simulink model "v2021_10_27_modello_calcolo_trim_1"  (R2020b)
settings: Solver=ode4  StartTime=0.0  StopTime=10  FixedStep=0.01  RelTol=1e-3
values from neighbouring files (symbols this model uses):
  alphavec_rad = [-0.10471975512 -0.0872664625997 -0.0698131700798 -0.0523598775598 -0.0349065850399 -0.0174532925199 0 0.0174532925199 0.0349065850399 0.0523598775598 0.0698131700798 0.0872664625997 ... (13 elements, 1x13)]    [datiAerodinamiciAENEA.mat]    (also in v2021_10_27_calcoloAerodinamica.m = deg2rad(alphavec))
  b = 2.62    [datiAerodinamiciAENEA.mat]    (also in derivateROSKAM_new.m; v2021_10_27_calcoloAerodinamica.m)
  betavec_rad = [-0.209439510239 -0.13962634016 -0.0698131700798 0 0.0698131700798 0.13962634016 0.209439510239]    [datiAerodinamiciAENEA.mat]    (also in v2021_10_27_calcoloAerodinamica.m = deg2rad(betavec))
  c = 0.32    [datiAerodinamiciAENEA.mat]    (also in derivateROSKAM_new.m; v2021_10_27_calcoloAerodinamica.m)
  cbar = 0.32    [datiAerodinamiciAENEA.mat]    (also in v2021_10_27_calcoloAerodinamica.m)
  CD0 = 0.2    [datiAerodinamiciAENEA.mat]    (also in v2021_10_27_calcoloAerodinamica.m = 0.024)
  CldA = KCldA(1)*180/pi    [Alettoni.m]    (also in datiAerodinamiciAENEA.mat = 0.490103315517)
  CLdE = KCLdE(1)*180/pi    [Equilibratore.m]    (also in datiAerodinamiciAENEA.mat = 0.809101149087)
  CldR = 0.0568697125654    [datiAerodinamiciAENEA.mat]
  Clp = -0.4318    [datiAerodinamiciAENEA.mat]    (also in derivateROSKAM_new.m = clp_w+2*(Zv/b)^2*cy_betav+Clp_tail; v2021_10_27_calcoloAerodinamica.m)
  CLq = 8.13    [datiAerodinamiciAENEA.mat]    (also in v2021_10_27_calcoloAerodinamica.m)
  Clr = 0.1459    [datiAerodinamiciAENEA.mat]    (also in derivateROSKAM_new.m = cl*clr_cl-(2/b^2)*(lv*cos(alpha)+Zv*sin(alpha))*(Zv*cos(alph; v2021_10_27_calcoloAerodinamica.m)
  CmdE = KCmdE(1)*180/pi    [Equilibratore.m]    (also in datiAerodinamiciAENEA.mat = -3.59730623976)
  Cmq = -23.24    [datiAerodinamiciAENEA.mat]    (also in derivateROSKAM_new.m = -K*cL_alphaw*((AR*(2*(Xw/c)^2+0.5*(Xw/c))/(AR+2))+1/8)-2*cL_; v2021_10_27_calcoloAerodinamica.m)
  CndA = KCndA(1)*180/pi    [Alettoni.m]    (also in datiAerodinamiciAENEA.mat = -0.0456969018066)
  CndR = -0.162544523826    [datiAerodinamiciAENEA.mat]
  Cnp = 0.000294    [datiAerodinamiciAENEA.mat]    (also in derivateROSKAM_new.m = -clp_w*tan(alpha)+Clp*tan(alpha)-(2/b)*(lv*cos(alpha)+Zv*sin; v2021_10_27_calcoloAerodinamica.m = 0.007507)
  Cnr = -0.4872    [datiAerodinamiciAENEA.mat]    (also in derivateROSKAM_new.m = (Cnr_Clquadro)*cl^2+(cnr_cd0)*cd0+(2/b^2)*(lv*cos(alpha)+Zv*; v2021_10_27_calcoloAerodinamica.m)
  CYdA = KCYdA(1)*180/pi    [Alettoni.m]    (also in datiAerodinamiciAENEA.mat = -0.0146577407549)
  CYdR = -0.298131751664    [datiAerodinamiciAENEA.mat]
  CYp = 0.050728    [datiAerodinamiciAENEA.mat]    (also in v2021_10_27_calcoloAerodinamica.m)
  CYr = 0.358925    [datiAerodinamiciAENEA.mat]    (also in v2021_10_27_calcoloAerodinamica.m)
  deltaAtrim = 0    [v2021_10_27_avvioSITL.m]
  deltaEtrim = (Cm0*CL_alpharad+Cm_alpharad*CLtrim)/(CL_alpharad*CmdE)    [calcoloDatiIniziali.m]    (also in v2021_10_27_avvioSITL.m = 0)
  deltaRtrim = 0    [v2021_10_27_avvioSITL.m]
  deltaTtrim = 0.1    [v2021_10_27_avvioSITL.m]
  Dprop = 0.5334    [datiAerodinamiciAENEA.mat]    (also in v2021_10_27_calcoloAerodinamica.m)
  J_vec = [0 0.03 0.06 0.09 0.11 0.14 0.17 0.2 0.23 0.26 0.28 0.31 ... (30 elements, 30x1)]    [datiAerodinamiciAENEA.mat]
  Jeng = 0    [datiAerodinamiciAENEA.mat]    (also in v2021_10_27_calcoloAerodinamica.m)
  Jprop = 0.00422031414    [datiAerodinamiciAENEA.mat]    (also in v2021_10_27_calcoloAerodinamica.m)
  q = prediction(11)    [f_pred_F1B.m]
  r = prediction(12)    [f_pred_F1B.m]
  rACtG = [-1.334 0 -0.2103]    [datiAerodinamiciAENEA.mat]    (also in v2021_10_27_calcoloAerodinamica.m = rACtP-rGP)
  rACwG = [-0.0589 0 -0.1645]    [datiAerodinamiciAENEA.mat]    (also in v2021_10_27_calcoloAerodinamica.m = rACwP-rGP)
  rAHRSG = [0 0 0.1075]    [datiAerodinamiciAENEA.mat]    (also in v2021_10_27_calcoloAerodinamica.m = rAHRSP-rGP)
  rho = 1.2133    [datiAerodinamiciAENEA.mat]    (also in derivateROSKAM_new.m = 1.16123787958; v2021_10_27_calcoloAerodinamica.m)
  rLEG = [0.0211 0 -0.1645]    [datiAerodinamiciAENEA.mat]    (also in v2021_10_27_calcoloAerodinamica.m = rLEP-rGP)
  rmglG = [-0.2319 -0.2 0.3925]    [datiAerodinamiciAENEA.mat]    (also in v2021_10_27_calcoloAerodinamica.m = rmglP-rGP)
  rmgrG = [-0.2319 0.2 0.3925]    [datiAerodinamiciAENEA.mat]    (also in v2021_10_27_calcoloAerodinamica.m = rmgrP-rGP)
  rngG = [0.2969 0 0.3925]    [datiAerodinamiciAENEA.mat]    (also in v2021_10_27_calcoloAerodinamica.m = rngP-rGP)
  rNPG = [-0.2442 0 -0.1645]    [datiAerodinamiciAENEA.mat]    (also in v2021_10_27_calcoloAerodinamica.m = rNPP-rGP)
  rPG = [0.5 0 -0.1075]    [datiAerodinamiciAENEA.mat]    (also in v2021_10_27_calcoloAerodinamica.m = -rGP)
  Rprop = 0.2667    [datiAerodinamiciAENEA.mat]    (also in v2021_10_27_calcoloAerodinamica.m)
  S = 0.8384    [datiAerodinamiciAENEA.mat]    (also in derivateROSKAM_new.m; v2021_10_27_calcoloAerodinamica.m)
  W = [0 0 92.214]    [datiAerodinamiciAENEA.mat]    (also in derivateROSKAM_new.m = 112.815; v2021_10_27_calcoloAerodinamica.m = m*g)
  Zeng = -0.1075    [datiAerodinamiciAENEA.mat]    (also in v2021_10_27_calcoloAerodinamica.m = rPG(3))
undefined symbols (not defined in the file or in its folder): F, matricepolinomi, MIL
libraries: aerolibwind2 x3, simulink x2, shared6dof x1, aerolibasang x1, pid_lib x1
(part 2 of 2)

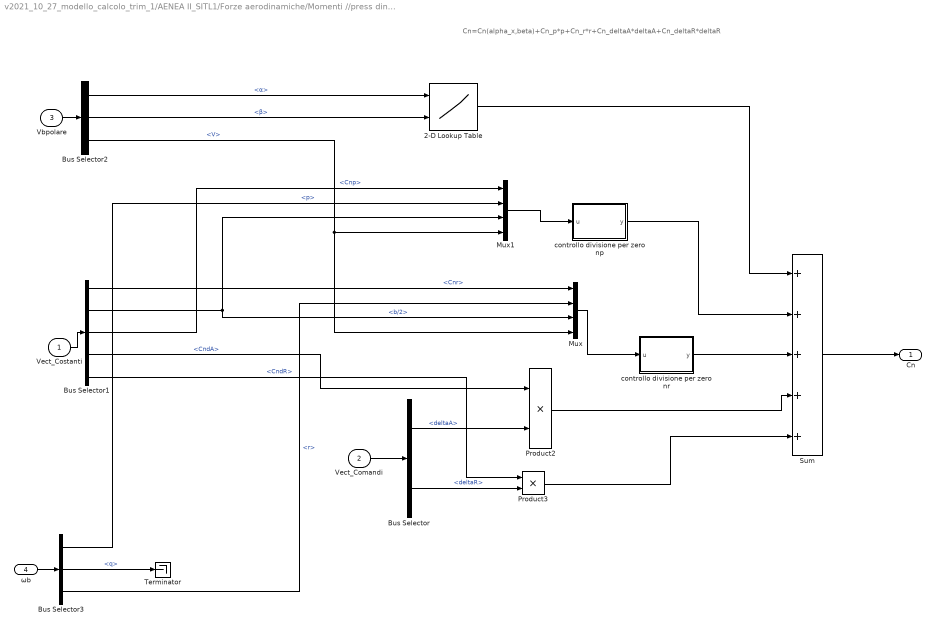
== system v2021_10_27_modello_calcolo_trim_1/AENEA II_SITL1/Forze aerodinamiche/Momenti //press din/Subsystem5 ==
  note: Cn=Cn(alpha_x,beta)+Cn_p*p+Cn_r*r+Cn_deltaA*deltaA+Cn_deltaR*deltaR
  Vect_Costanti : Inport
  Vect_Comandi : Inport  Port=2
  "Vbpolare " : Inport  Port=3
  ωb : Inport  Port=4
  2-D Lookup Table : Lookup_n-D  BreakpointsForDimension1=alphavec_rad  BreakpointsForDimension2=betavec_rad  Table=Cn(2:end,2:end)  InternalRulePriority=Speed  RndMeth=Simplest  InputSameDT=on
      settings: InputPortMap=u0,u1
  Bus Selector : BusSelector  OutputSignals=deltaA,deltaR
  Bus Selector1 : BusSelector  OutputSignals=Coef_Aerodinamici.Coef_Momenti.Cnr,Coef_Geometrici.b/2,Coef_Aerodinamici.Coef_Momenti.Cnp,Coef_Aerodinamici.Coef_Momenti.CndA,Coef_Aerodinamici.Coef_Momenti.CndR
  Bus Selector2 : BusSelector  OutputSignals=α,β,V
  Bus Selector3 : BusSelector  OutputSignals=p,q,r
  Mux : Mux
  Mux1 : Mux
  Product2 : Product
  Product3 : Product
  Sum : Sum  Inputs=5
  Terminator : Terminator
  "controllo divisione per zero np " : MATLAB Function  TreatAsAtomicUnit=on
  "controllo divisione per zero nr " : MATLAB Function  TreatAsAtomicUnit=on
  Cn : Outport  VectorParamsAs1DForOutWhenUnconnected=off
  wires:
  Bus Selector1/3 -> Mux1/1  "<Cnp>"
  Product2/1 -> Sum/4
  Product3/1 -> Sum/5
  Sum/1 -> Cn/1
  Bus Selector1/1 -> Mux/1  "<Cnr>"
  Bus Selector1/5 -> Product3/1  "<CndR>"
  Bus Selector/2 -> Product3/2  "<deltaR>"
  Bus Selector/1 -> Product2/2  "<deltaA>"
  2-D Lookup Table/1 -> Sum/1
  Vect_Comandi/1 -> Bus Selector/1
  Vect_Costanti/1 -> Bus Selector1/1
  Bus Selector1/4 -> Product2/1  "<CndA>"
  Bus Selector1/2 -> Mux1/3, Mux/3  "<b/2>"
  Bus Selector2/3 -> Mux1/4, Mux/4  "<V>"
  "Vbpolare "/1 -> Bus Selector2/1
  Bus Selector2/1 -> 2-D Lookup Table/1  "<α>"
  Bus Selector2/2 -> 2-D Lookup Table/2  "<β>"
  ωb/1 -> Bus Selector3/1
  Bus Selector3/3 -> Mux/2  "<r>"
  Bus Selector3/1 -> Mux1/2  "<p>"
  Bus Selector3/2 -> Terminator/1  "<q>"
  Mux/1 -> "controllo divisione per zero nr "/1(u)
  "controllo divisione per zero nr "/1(y) -> Sum/3
  Mux1/1 -> "controllo divisione per zero np "/1(u)
  "controllo divisione per zero np "/1(y) -> Sum/2

== matlab function v2021_10_27_modello_calcolo_trim_1/AENEA II_SITL1/Velocità1/MATLAB Function ==
  data: V input; module output
function module = absolute(V)

module=sqrt((V(1)^2)+(V(2)^2)+(V(3)^2));

end

== matlab function v2021_10_27_modello_calcolo_trim_1/AENEA II_SITL1/Velocità1/controllo divisione per 0 su alpha ==
  data: u input; y output
function y = tgalpha(u)

if length(u)~=2
    error('vettore ingresso errato')
else
    if u(2)==0
        y=0;
    else 
        y=u(1)/u(2);
    end
end

== matlab function v2021_10_27_modello_calcolo_trim_1/AENEA II_SITL1/Velocità1/controllo divisione per 0 su beta ==
  data: u input; y output
function y = sinbeta(u)

if length(u)~=2
    error('vettore ingresso errato')
else
    if u(2)==0
        y=0;
    else 
        y=u(1)/u(2);
    end
end

== matlab function v2021_10_27_modello_calcolo_trim_1/AENEA II_SITL1/Velocità1/MATLAB Function1 ==
  data: V input; module output
function module = absolute(V)

module=sqrt((V(1)^2)+(V(2)^2)+(V(3)^2));

end

== matlab function v2021_10_27_modello_calcolo_trim_1/AENEA II_SITL1/Forze aerodinamiche/Forze assi vento//q/Subsystem1/controllo divisione per zero Yp  ==
  data: u input; y output
function y = Yp(u)

if length(u)~=4
    error('vettore ingresso dimensione errata')
else
    if u(4)==0
        y=0;
    else
        y=u(1)*u(2)*u(3)/u(4);
    end
end

== matlab function v2021_10_27_modello_calcolo_trim_1/AENEA II_SITL1/Forze aerodinamiche/Forze assi vento//q/Subsystem1/controllo divisione per zero Yr ==
  data: u input; y output
function y = Yr(u)

if length(u)~=4
    error('vettore ingresso dimensione errata')
else
    if u(4)==0
        y=0;
    else
        y=u(1)*u(2)*u(3)/u(4);
    end
end

== matlab function v2021_10_27_modello_calcolo_trim_1/AENEA II_SITL1/Forze aerodinamiche/Forze assi vento//q/Subsystem2/controllo divisione per zero Lq  ==
  data: u input; y output
function y = Lq(u)

if length(u)~=4
    error('vettore ingresso dimensione errata')
else
    if u(4)==0
        y=0;
    else
        y=u(1)*u(2)*u(3)/u(4);
    end
end

== matlab function v2021_10_27_modello_calcolo_trim_1/AENEA II_SITL1/Forze aerodinamiche/MATLAB Function ==
  data: alpha input; Lbw output; beta input
function Lbw = DCMbw(alpha,beta)


Lbw=[cos(alpha)*cos(beta), -cos(alpha)*sin(beta), -sin(alpha); sin(beta), cos(beta), 0; sin(alpha)*cos(beta), -sin(alpha)*sin(beta), cos(alpha)];

== matlab function v2021_10_27_modello_calcolo_trim_1/AENEA II_SITL1/Forze aerodinamiche/Momenti //press din/Subsystem3/controllo divisione per zero lp  ==
  data: u input; y output
function y = lp(u)

if length(u)~=4
    error('vettore ingresso dimensione errata')
else
    if u(4)==0
        y=0;
    else
        y=u(1)*u(2)*u(3)/u(4);
    end
end

== matlab function v2021_10_27_modello_calcolo_trim_1/AENEA II_SITL1/Forze aerodinamiche/Momenti //press din/Subsystem3/controllo divisione per zero lr  ==
  data: u input; y output
function y = lr(u)

if length(u)~=4
    error('vettore ingresso dimensione errata')
else
    if u(4)==0
        y=0;
    else
        y=u(1)*u(2)*u(3)/u(4);
    end
end

== matlab function v2021_10_27_modello_calcolo_trim_1/AENEA II_SITL1/Forze aerodinamiche/Momenti //press din/Subsystem4/controllo divisione per zero mq  ==
  data: u input; y output
function y = mq(u)

if length(u)~=4
    error('vettore ingresso dimensione errata')
else
    if u(4)==0
        y=0;
    else
        y=u(1)*u(2)*u(3)/u(4);
    end
end

== matlab function v2021_10_27_modello_calcolo_trim_1/AENEA II_SITL1/Forze aerodinamiche/Momenti //press din/Subsystem5/controllo divisione per zero np  ==
  data: u input; y output
function y = np(u)

if length(u)~=4
    error('vettore ingresso dimensione errata')
else
    if u(4)==0
        y=0;
    else
        y=u(1)*u(2)*u(3)/u(4);
    end
end

== matlab function v2021_10_27_modello_calcolo_trim_1/AENEA II_SITL1/Forze aerodinamiche/Momenti //press din/Subsystem5/controllo divisione per zero nr  ==
  data: u input; y output
function y = nr(u)

if length(u)~=4
    error('vettore ingresso dimensione errata')
else
    if u(4)==0
        y=0;
    else
        y=u(1)*u(2)*u(3)/u(4);
    end
end

== matlab function v2021_10_27_modello_calcolo_trim_1/AENEA II_SITL1/MATLAB Function ==
  data: PHI input; invR output
function invR = omega2PHIdot(PHI)

if length(PHI)==3
    Phi=PHI(1);
    Theta=PHI(2);
    
    invR=[1, sin(Phi)*tan(Theta), cos(Phi)*tan(Theta); 0, cos(Phi), -sin(Phi); 0, sin(Phi)*sec(Theta), cos(Phi)*sec(Theta)];
else 
    error('il vettore PHI non va bene')
end

== matlab function v2021_10_27_modello_calcolo_trim_1/AENEA II_SITL1/Propulsione1/LUT ELICA /MATLAB Function ==
  data: J input; Ct output; RPM input; Cp output; matricepolinomi input
function [Ct,Cp] = calcolo_Ct_Cp(J,RPM,matricepolinomi)

lct00 = matricepolinomi(1,1);
lct10 = matricepolinomi(1,2);
lct01 = matricepolinomi(1,3);
lct20 = matricepolinomi(1,4);
lct11 = matricepolinomi(1,5);
lct02 = matricepolinomi(1,6);
lct30 = matricepolinomi(1,7);
lct21 = matricepolinomi(1,8);
lct12 = matricepolinomi(1,9);
lct40 = matricepolinomi(1,10);
lct31 = matricepolinomi(1,11);
lct22 = matricepolinomi(1,12);

qct00 = matricepolinomi(2,1);
qct10 = matricepolinomi(2,2);
qct01 = matricepolinomi(2,3);
qct20 = matricepolinomi(2,4);
qct11 = matricepolinomi(2,5);
qct02 = matricepolinomi(2,6);
qct30 = matricepolinomi(2,7);
qct21 = matricepolinomi(2,8);
qct12 = matricepolinomi(2,9);
qct03 = matricepolinomi(2,10);
qct40 = matricepolinomi(2,11);
qct31 = matricepolinomi(2,12);
qct22 = matricepolinomi(2,13);
qct13 = matricepolinomi(2,14);
qct04 = matricepolinomi(2,15);
qct50 = matricepolinomi(2,16);
qct41 = matricepolinomi(2,17);
qct32 = matricepolinomi(2,18);
qct23 = matricepolinomi(2,19);
qct14 = matricepolinomi(2,20);
qct05 = matricepolinomi(2,21);

cp100 = matricepolinomi(3,1);
cp110 = matricepolinomi(3,2);
cp101 = matricepolinomi(3,3);
cp120 = matricepolinomi(3,4);
cp111 = matricepolinomi(3,5);
cp102 = matricepolinomi(3,6);
cp130 = matricepolinomi(3,7);
cp121 = matricepolinomi(3,8);
cp112 = matricepolinomi(3,9);
cp140 = matricepolinomi(3,10);
cp131 = matricepolinomi(3,11);
cp122 = matricepolinomi(3,12);

cp200 = matricepolinomi(4,1);
cp210 = matricepolinomi(4,2);
cp201 = matricepolinomi(4,3);
cp220 = matricepolinomi(4,4);
cp211 = matricepolinomi(4,5);
cp202 = matricepolinomi(4,6);
cp230 = matricepolinomi(4,7);
cp221 = matricepolinomi(4,8);
cp212 = matricepolinomi(4,9);
cp240 = matricepolinomi(4,10);
cp231 = matricepolinomi(4,11);
cp222 = matricepolinomi(4,12);

cp300 = matricepolinomi(5,1);
cp310 = matricepolinomi(5,2);
cp301 = matricepolinomi(5,3);
cp320 = matricepolinomi(5,4);
cp311 = matricepolinomi(5,5);
cp302 = matricepolinomi(5,6);
cp330 = matricepolinomi(5,7);
cp321 = matricepolinomi(5,8);
cp312 = matricepolinomi(5,9);
cp340 = matricepolinomi(5,10);
cp331 = matricepolinomi(5,11);
cp322 = matricepolinomi(5,12);

cp400 = matricepolinomi(6,1);
cp410 = matricepolinomi(6,2);
cp401 = matricepolinomi(6,3);
cp420 = matricepolinomi(6,4);
cp411 = matricepolinomi(6,5);
cp402 = matricepolinomi(6,6);
cp430 = matricepolinomi(6,7);
cp421 = matricepolinomi(6,8);
cp412 = matricepolinomi(6,9);
cp440 = matricepolinomi(6,10);
cp431 = matricepolinomi(6,11);
cp422 = matricepolinomi(6,12);


if J<=0.32
    x = RPM;
    y = J;
    Ct = qct00 + qct10*x + qct01*y + qct20*x^2 + qct11*x*y + qct02*y^2 + qct30*x^3 + qct21*x^2*y + qct12*x*y^2 + qct03*y^3 + qct40*x^4 + qct31*x^3*y + qct22*x^2*y^2 + qct13*x*y^3 + qct04*y^4 + qct50*x^5 + qct41*x^4*y + qct32*x^3*y^2 + qct23*x^2*y^3 + qct14*x*y^4 + qct05*y^5;
elseif J>0.32
    x = RPM;
    y = J;
    Ct = lct00 + lct10*x + lct01*y + lct20*x^2 + lct11*x*y + lct02*y^2 + lct30*x^3 + lct21*x^2*y + lct12*x*y^2 + lct40*x^4 + lct31*x^3*y + lct22*x^2*y^2;
else
    Ct = 0;
end

if (J<=0.34)&&(RPM<=5000)
    x = RPM;
    y = J;
    Cp = cp100 + cp110*x + cp101*y + cp120*x^2 + cp111*x*y + cp102*y^2 + cp130*x^3 + cp121*x^2*y + cp112*x*y^2 + cp140*x^4 + cp131*x^3*y + cp122*x^2*y^2;
elseif (J<=0.34)&&(RPM>5000)
    x = RPM;
    y = J;
    Cp = cp200 + cp210*x + cp201*y + cp220*x^2 + cp211*x*y + cp202*y^2 + cp230*x^3 + cp221*x^2*y + cp212*x*y^2 + cp240*x^4 + cp231*x^3*y + cp222*x^2*y^2;
elseif (J>0.34)&&(RPM<=5000)
    x = RPM;
    y = J;
    Cp = cp300 + cp310*x + cp301*y + cp320*x^2 + cp311*x*y + cp302*y^2 + cp330*x^3 + cp321*x^2*y + cp312*x*y^2 + cp340*x^4 + cp331*x^3*y + cp322*x^2*y^2;
elseif (J>0.34)&&(RPM>5000)
    x = RPM;
    y = J;
    Cp = cp400 + cp410*x + cp401*y + cp420*x^2 + cp411*x*y + cp402*y^2 + cp430*x^3 + cp421*x^2*y + cp412*x*y^2 + cp440*x^4 + cp431*x^3*y + cp422*x^2*y^2;
else
    Cp = 0;
end
